simulink model "modele_lqr"  (R2026a)
settings: Solver=VariableStepAuto
values from neighbouring files (symbols this model uses):
  A_obs = A - L*C    [init_lqr.m]
  B_obs = [B, L]    [init_lqr.m]
  C_obs = eye(4)    [init_lqr.m]
  D_obs = zeros(4,3)    [init_lqr.m]
  g = 9.81    [init_params.m]
  K = lqr(A, B, Q, R)    [init_lqr.m]
  l = 0.5    [init_params.m]
  M = 1.0    (= 1)    [init_params.m]
  m = 0.1    [init_params.m]
  theta0 = pi*theta0/180    (= 0.174532925199)    [init_params.m]
libraries: simulink x1
settings Model: Creator=floberg  LastModifiedBy=floberg

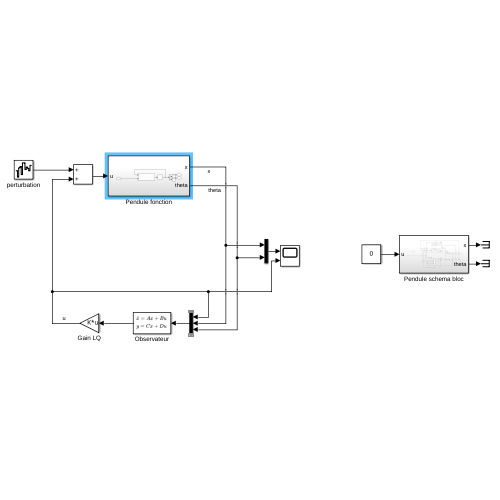
[thumbnail: Simulink's stored preview of the top-level diagram]
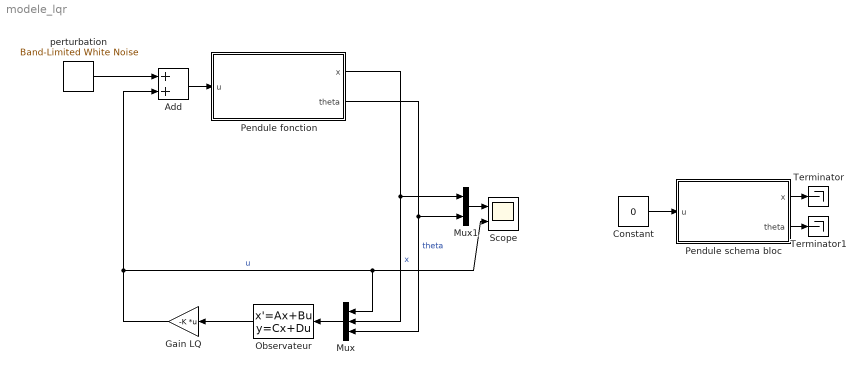
== system modele_lqr ==
  Add : Sum
  Constant : Constant  Value=0
  Gain LQ : Gain  Gain=-K  Multiplication=Matrix(K*u)
  Mux : Mux  Inputs=3
  Mux1 : Mux  Inputs=2
  Observateur : StateSpace  A=A_obs  B=B_obs  C=C_obs  D=D_obs  InitialCondition=0
  Pendule fonction : Subsystem
  Pendule schema bloc : Subsystem
  Scope : Scope  NumInputPorts=2
      settings: ActiveDisplayYMinimum=-0.21417856701218485  ActiveDisplayYMaximum=0.23818380454524826
  Terminator : Terminator
  Terminator1 : Terminator
  perturbation : simulink/Sources/Band-Limited White Noise  Cov=[1e-2]  Ts=1  seed=[23341]
  wires:
  Mux/1 -> Observateur/1
  Observateur/1 -> Gain LQ/1
  Gain LQ/1 -> Mux/1, Scope/2, Add/2  "u"
  Pendule fonction/2(theta) -> Mux/3, Mux1/2  "theta"
  Pendule fonction/1(x) -> Mux/2, Mux1/1  "x"
  Pendule schema bloc/1(x) -> Terminator/1
  Pendule schema bloc/2(theta) -> Terminator1/1
  Constant/1 -> Pendule schema bloc/1(u)
  perturbation/1 -> Add/1
  Add/1 -> Pendule fonction/1(u)
  Mux1/1 -> Scope/1

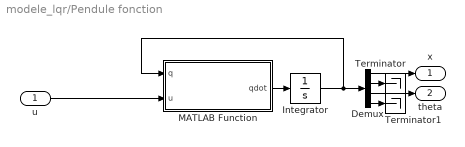
== system modele_lqr/Pendule fonction ==
  u : Inport
  Demux : Demux
  Integrator : Integrator  InitialCondition=[0;0;theta0;0]  UpperSaturationLimit=[100;100;6;100]  LowerSaturationLimit=[-100;-100;-6;-100]
  MATLAB Function : MATLAB Function  TreatAsAtomicUnit=on
  Terminator : Terminator
  Terminator1 : Terminator
  x : Outport
  theta : Outport  Port=2
  wires:
  Integrator/1 -> MATLAB Function/1(q), Demux/1
  Demux/3 -> theta/1
  MATLAB Function/1(qdot) -> Integrator/1
  Demux/1 -> x/1
  u/1 -> MATLAB Function/2(u)
  Demux/2 -> Terminator/1
  Demux/4 -> Terminator1/1

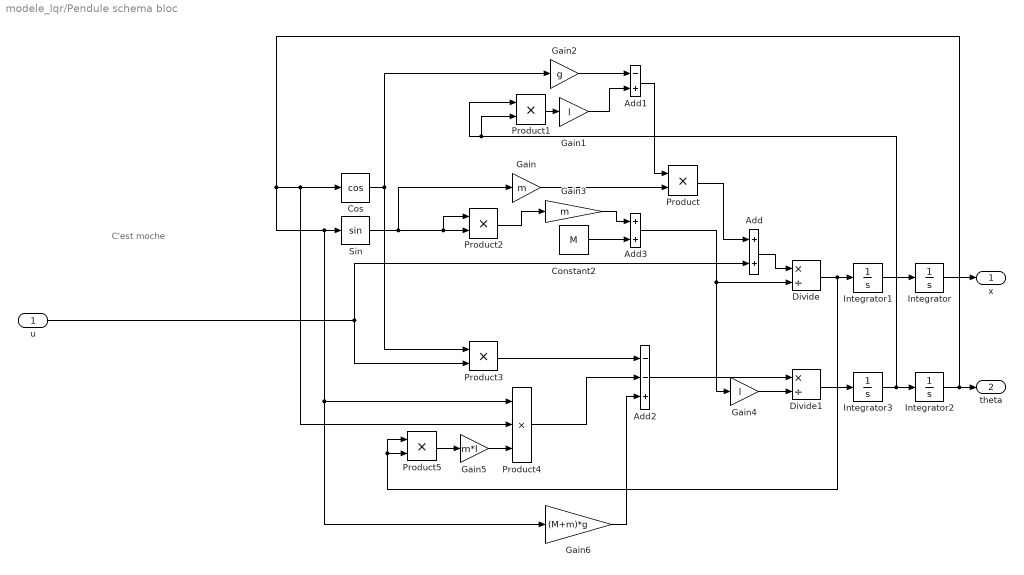
== system modele_lqr/Pendule schema bloc ==
  note: C'est moche
  u : Inport
  Add : Sum
  Add1 : Sum  Inputs=-+
  Add2 : Sum  Inputs=--+
  Add3 : Sum
  Constant2 : Constant  Value=M
  Cos : Trigonometry  Operator=cos
  Divide : Product  Inputs=*/
  Divide1 : Product  Inputs=*/
  Gain : Gain  Gain=m
  Gain1 : Gain  Gain=l
  Gain2 : Gain  Gain=g
  Gain3 : Gain  Gain=m
  Gain4 : Gain  Gain=l
  Gain5 : Gain  Gain=m*l
  Gain6 : Gain  Gain=(M+m)*g
  Integrator : Integrator
  Integrator1 : Integrator
  Integrator2 : Integrator  InitialCondition=theta0
  Integrator3 : Integrator
  Product{,1..3,5} (5 alike) : Product
  Product4 : Product  Inputs=3
  Sin : Trigonometry
  x : Outport
  theta : Outport  Port=2
  wires:
  Integrator/1 -> x/1
  Integrator1/1 -> Integrator/1
  Integrator3/1 -> Product1/1, Product1/2, Integrator2/1
  Integrator2/1 -> Product4/2, Cos/1, Gain6/1, Product4/1, Sin/1, theta/1
  Divide1/1 -> Integrator3/1
  Sin/1 -> Product2/2, Product2/1, Gain/1
  Gain/1 -> Product/2
  Product1/1 -> Gain1/1
  Gain2/1 -> Add1/1
  Cos/1 -> Gain2/1, Product3/1
  Product2/1 -> Gain3/1
  Gain3/1 -> Add3/1
  Product/1 -> Add/1
  Gain1/1 -> Add1/2
  Add1/1 -> Product/1
  u/1 -> Product3/2, Add/2
  Divide/1 -> Product5/2, Product5/1, Integrator1/1
  Add/1 -> Divide/1
  Add2/1 -> Divide1/1
  Product3/1 -> Add2/1
  Gain5/1 -> Product4/3
  Product5/1 -> Gain5/1
  Product4/1 -> Add2/2
  Gain6/1 -> Add2/3
  Constant2/1 -> Add3/2
  Add3/1 -> Gain4/1, Divide/2
  Gain4/1 -> Divide1/2

== matlab function modele_lqr/Pendule fonction/MATLAB Function ==
  data: q input; u input; qdot output
function qdot = pendule_nonlineaire(q, u)
    % Paramètres
    M = 1.0; m = 0.1; l = 0.5; g = 9.81;

    x     = q(1);
    xdot  = q(2);
    theta = q(3);
    tdot  = q(4);  % theta_dot

    D = M + m*sin(theta)^2; % Dénominateur commun

    % Equations exactes non linéaires
    xddot = ( u + m*sin(theta)*(l*tdot^2 - g*cos(theta)) ) / D;

    tddot = ( -u*cos(theta) ...
              - m*l*tdot^2*sin(theta)*cos(theta) ...
              + (M+m)*g*sin(theta) ) / (l * D);

    qdot = [xdot; xddot; tdot; tddot];
end
